simulink model "si4_forcedspringmassdamper"  (R2023b)
settings: Solver=VariableStepAuto  StartTime=0.0  StopTime=te  RelTol=1e-3
values from neighbouring files (symbols this model uses):
  c = -0.8    [si5_Ball_parameter.m]    (also in sim21_ODE.m = 1)
  F = 1    [sim21_ODE.m]
  k = 10    [si5_Ball_parameter.m]    (also in sim21_ODE.m = 3)
  m = 0.35    [Electromagnet_par.m]    (also in si5_Ball_parameter.m = 0.1; sim21_ODE.m = 3)
  w = 2*pi/0.1    (= 62.8318530718)    [Electromagnet_par.m]    (also in coil_ironcore.m = 314.159265359; sim21_ODE.m = [0.5 1 2])
settings Model: Creator=sar  LastModifiedBy=sar

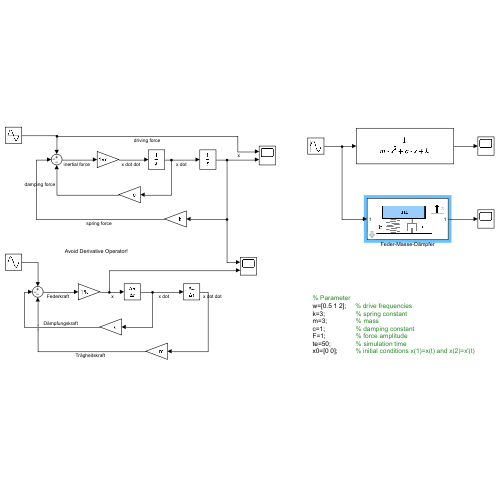
[thumbnail: Simulink's stored preview of the top-level diagram]
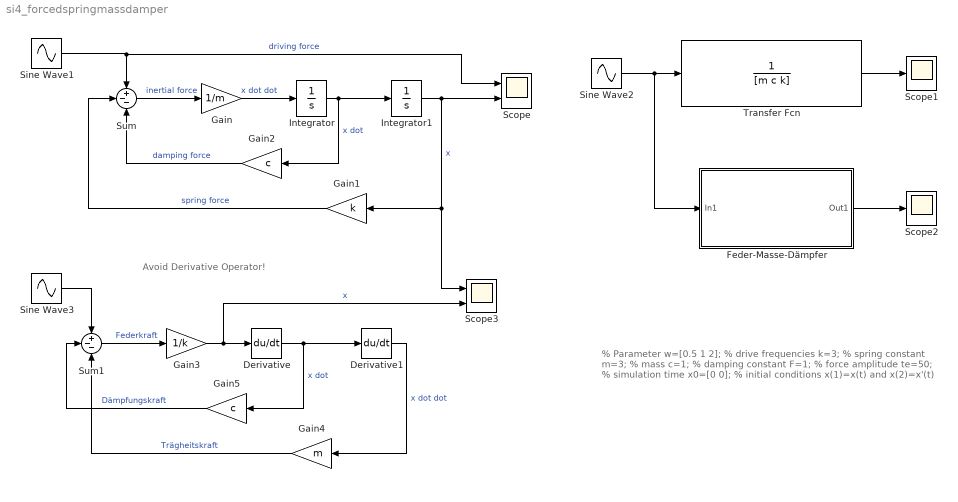
== system si4_forcedspringmassdamper ==
  note: Avoid Derivative Operator!
  note: % Parameter
      | w=[0.5 1 2]; % drive frequencies
      | k=3; % spring constant
      | m=3; % mass
      | c=1; % damping constant
      | F=1; % force amplitude
      | te=50; % simulation time
      | x0=[0 0]; % initial conditions x(1)=x(t) and x(2)=x'(t)
  Derivative : Derivative
  Derivative1 : Derivative
  Feder-Masse-Dämpfer : Subsystem  mask{m=m, k=k, c=c}
      mask prompts: m "Masse"; k "Federsteifigkeit"; c "Daempfungskonstante"
      mask Display: image('simulink/si4_mass_spring_damper.png');
  Gain : Gain  Gain=1/m
  Gain1 : Gain  Gain=k
  Gain2 : Gain  Gain=c
  Gain3 : Gain  Gain=1/k
  Gain4 : Gain  Gain=m
  Gain5 : Gain  Gain=c
  Integrator : Integrator
  Integrator1 : Integrator
  Scope : Scope  NumInputPorts=2
  Scope1 : Scope
  Scope2 : Scope
  Scope3 : Scope  NumInputPorts=2
  Sine Wave1 : Sin  Amplitude=F  Frequency=w  SampleTime=0
  Sine Wave2 : Sin  Amplitude=F  Frequency=w(2)  SampleTime=0
  Sine Wave3 : Sin  Amplitude=F  Frequency=w  SampleTime=0
  Sum : Sum  Inputs=+--
  Sum1 : Sum  Inputs=+--
  Transfer Fcn : TransferFcn  Denominator=[m c k]
  wires:
  Integrator/1 -> Gain2/1, Integrator1/1  "x dot"
  Gain5/1 -> Sum1/2  "Dämpfungskraft"
  Derivative/1 -> Gain5/1, Derivative1/1  "x dot"
  Gain3/1 -> Scope3/2, Derivative/1  "x"
  Sum1/1 -> Gain3/1  "Federkraft"
  Sine Wave3/1 -> Sum1/1
  Gain4/1 -> Sum1/3  "Trägheitskraft"
  Derivative1/1 -> Gain4/1  "x dot dot"
  Sine Wave2/1 -> Feder-Masse-Dämpfer/1(In1), Transfer Fcn/1
  Feder-Masse-Dämpfer/1(Out1) -> Scope2/1
  Transfer Fcn/1 -> Scope1/1
  Sum/1 -> Gain/1  "inertial force"
  Gain/1 -> Integrator/1  "x dot dot"
  Sine Wave1/1 -> Scope/1, Sum/1  "driving force"
  Gain2/1 -> Sum/3  "damping force"
  Integrator1/1 -> Scope/2, Scope3/1, Gain1/1  "x"
  Gain1/1 -> Sum/2  "spring force"

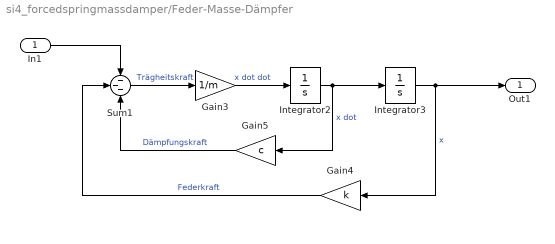
== system si4_forcedspringmassdamper/Feder-Masse-Dämpfer ==
  In1 : Inport
  Gain3 : Gain  Gain=1/m
  Gain4 : Gain  Gain=k
  Gain5 : Gain  Gain=c
  Integrator2 : Integrator
  Integrator3 : Integrator
  Sum1 : Sum  Inputs=---
  Out1 : Outport  VectorParamsAs1DForOutWhenUnconnected=off
  wires:
  Sum1/1 -> Gain3/1  "Trägheitskraft"
  Gain5/1 -> Sum1/3  "Dämpfungskraft"
  Gain3/1 -> Integrator2/1  "x dot dot"
  Integrator3/1 -> Out1/1, Gain4/1  "x"
  Gain4/1 -> Sum1/2  "Federkraft"
  Integrator2/1 -> Gain5/1, Integrator3/1  "x dot"
  In1/1 -> Sum1/1
